simulink model "AerialManipulatorControl"  (Simulink 8.8)
settings: Solver=FixedStepAuto  StartTime=0.0  StopTime=1  RelTol=1e-3
libraries: aerolib6dof2 x1, AerialManipulation x1
settings Model: Creator=Administrator  LastModifiedBy=Administrator
settings DataIOCC: LimitDataPoints=off  SaveFormat=Dataset  SignalLoggingSaveFormat=Dataset
settings OptimizationCC: LifeSpan=auto
settings DebuggingCC: UnderspecifiedInitializationDetection=Simplified  MergeDetectMultiDrivingBlocksExec=error  FcnCallInpInsideContextMsg=error  StateNameClashWarn=none  SFUnexpectedBacktrackingDiag=error  SFNoUnconditionalDefaultTransitionDiag=error  SFExecutionAtInitializationDiag=warning
settings HardwareCC: ProdBitPerPointer=64  ProdBitPerSizeT=64  ProdBitPerPtrDiffT=64  ProdLargestAtomicFloat=Float  ProdIntDivRoundTo=Zero  ProdEndianess=LittleEndian  ProdWordSize=64  ProdHWDeviceType=Intel->x86-64 (Windows64)
settings ModelReferenceCC: PropagateSignalLabelsOutOfModel=on
settings GRTTargetCC: TargetLangStandard=C99 (ISO)  GeneratePreprocessorConditionals=Use local settings  CombineOutputUpdateFcns=on  GRTInterface=off
settings ConfigComp: CovMetricSettings=dwe  CovHtmlReporting=off  CovSaveCumulativeToWorkspaceVar=off  CovSaveSingleToWorkspaceVar=off  CovExternalEMLEnable=on

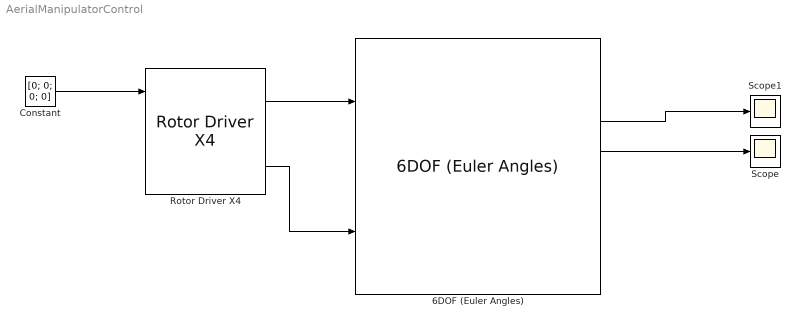
== system AerialManipulatorControl ==
  6DOF (Euler Angles) : aerolib6dof2/6DOF (Euler Angles)  units=Metric (MKS)  mtype=Fixed  rep=Euler Angles  xme_0=[0 0 0]  Vm_0=[0 0 0]  eul_0=[0 0 0.88]  pm_0=[0 0 0]  mass_0=1.0  mass_e=0.5  mass_f=2.0  inertia=eye(3)  inertia_e=eye(3)  inertia_f=2*eye(3)  k_quat=1.0  vre_flag=on
  Constant : Constant  Value=[0; 0; 0; 0]
  Rotor Driver X4 : AerialManipulation/Rotor Driver X4  l=0.18  Fe=[ [0;0;1],[0;0;1],[0;0;1],[0;0;1] ]  r=[ [0.18;0;0],[0;0.18;0],[-0.18;0;0],[0;-0.18;0] ]  Td=[ [0;0;1], [0;0;-1],[0;0;1],[0;0;-1] ]  Kct=3.16e-05  Ktf=0.01
  Scope : Scope
  Scope1 : Scope
  wires:
  6DOF (Euler Angles)/4 -> Scope/1
  6DOF (Euler Angles)/3 -> Scope1/1
  Constant/1 -> Rotor Driver X4/1
  Rotor Driver X4/1 -> 6DOF (Euler Angles)/1
  Rotor Driver X4/2 -> 6DOF (Euler Angles)/2
